simulink model "VanDerPol"  (R2017a)
settings: Solver=FixedStepAuto  StartTime=0.0  StopTime=50.0  FixedStep=0.1  RelTol=1e-3
libraries: simulink x1
settings Model: Creator=Soutrik  LastModifiedBy=Soutrik

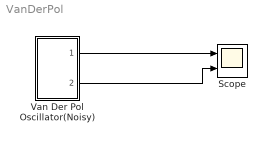
== system VanDerPol ==
  Scope : Scope  NumInputPorts=2
  Van Der Pol Oscillator(Noisy) : Subsystem
  wires:
  Van Der Pol Oscillator(Noisy)/1(State 1) -> Scope/1
  Van Der Pol Oscillator(Noisy)/2(State 2) -> Scope/2

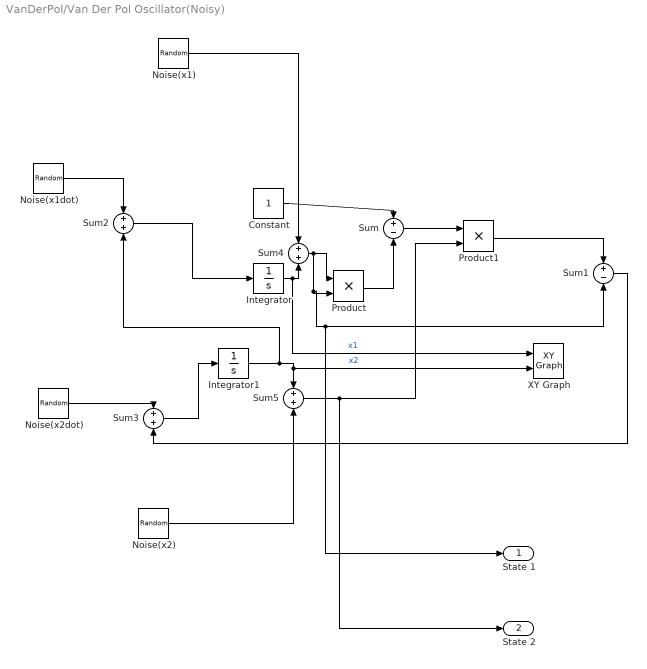
== system VanDerPol/Van Der Pol Oscillator(Noisy) ==
  Constant : Constant
  Integrator : Integrator  InitialCondition=0.1
  Integrator1 : Integrator  InitialCondition=0.1
  Noise(x1) : RandomNumber  Variance=0.015  Seed=73  SampleTime=0.1
  Noise(x1dot) : RandomNumber  Variance=0.2  Seed=43  SampleTime=0.1
  Noise(x2) : RandomNumber  Variance=0.025  Seed=87  SampleTime=0.1
  Noise(x2dot) : RandomNumber  Variance=0.1  Seed=57  SampleTime=0.1
  Product : Product
  Product1 : Product
  Sum : Sum  Inputs=+-
  Sum1 : Sum  Inputs=+-
  Sum{2..5} (4 alike) : Sum  Inputs=2
  XY Graph : simulink/Sinks/XY Graph  xmin=-3  xmax=3  ymin=-3  ymax=3  st=0.1
  State 1 : Outport
  State 2 : Outport  Port=2
  wires:
  Sum3/1 -> Integrator1/1
  Sum2/1 -> Integrator/1
  Constant/1 -> Sum/1
  Sum/1 -> Product1/1
  Product/1 -> Sum/2
  Noise(x2)/1 -> Sum5/2
  Noise(x1dot)/1 -> Sum2/1
  Sum4/1 -> State 1/1, Sum1/2, Product/2, Product/1
  Noise(x2dot)/1 -> Sum3/1
  Noise(x1)/1 -> Sum4/1
  Sum1/1 -> Sum3/2
  Product1/1 -> Sum1/1
  Integrator/1 -> XY Graph/1, Sum4/2  "x1"
  Integrator1/1 -> Sum2/2, Sum5/1, XY Graph/2  "x2"
  Sum5/1 -> State 2/1, Product1/2
